simulink model "parity1"  (R2021b)
settings: Solver=ode45  StartTime=0.0  StopTime=30  RelTol=1e-3  EnableMultiTasking=on
undefined symbols (not defined in the file): A, B, C, D, Ef, Ff, Hus, Vs
settings Model: Creator=ak  LastModifiedBy=user
settings SolverCC: AlgebraicLoopSolver=TrustRegion
settings DataIOCC: LimitDataPoints=on  SaveFormat=Array  ReturnWorkspaceOutputs=off
settings OptimizationCC: ExpressionDepthLimit=2147483647  LifeSpan=inf
settings DebuggingCC: UnderspecifiedInitializationDetection=Classic  MergeDetectMultiDrivingBlocksExec=none  SolverPrmCheckMsg=warning  StateNameClashWarn=warning  SFUnexpectedBacktrackingDiag=warning  SFNoUnconditionalDefaultTransitionDiag=warning  SFExecutionAtInitializationDiag=none  SFMachineParentedDataDiag=warning  ArithmeticOperatorsInVariantConditions=warning
settings HardwareCC: ProdBitPerPointer=32  ProdBitPerSizeT=32  ProdBitPerPtrDiffT=32  ProdLargestAtomicFloat=None  ProdIntDivRoundTo=Undefined  ProdEndianess=Unspecified  ProdWordSize=32  ProdHWDeviceType=32-bit Generic
settings ModelReferenceCC: PropagateSignalLabelsOutOfModel=off
settings SFSimCC: SimUseLocalCustomCode=off  CustomCodeUndefinedFunction=UseInterfaceOnly
settings RTWCC: RTWUseLocalCustomCode=off
settings CodeAppCC: StateflowObjectComments=on
settings GRTTargetCC: TargetLangStandard=C89/C90 (ANSI)
settings ConfigComp: CovMetricSettings=dw  CovSaveCumulativeToWorkspaceVar=on  CovSaveSingleToWorkspaceVar=on  CovExternalEMLEnable=off

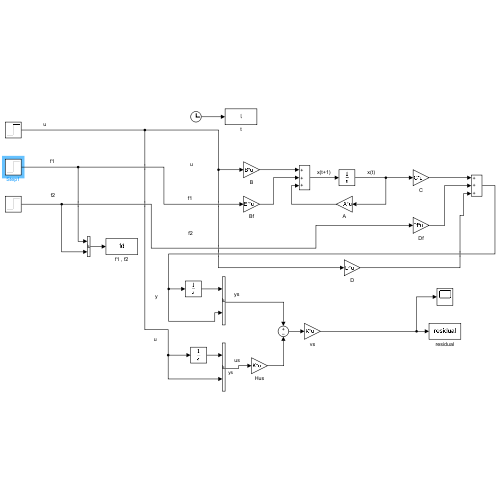
[thumbnail: Simulink's stored preview of the top-level diagram]
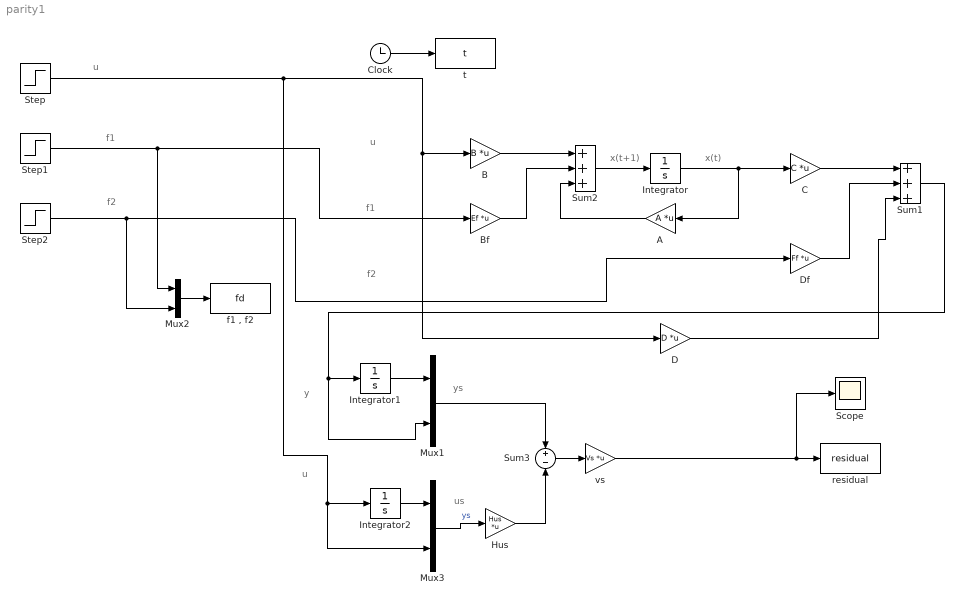
== system parity1 ==
  note: f2
  note: f1
  note: u
  note: x(t+1)
  note: f2
  note: f1
  note: x(t)
  note: u
  note: us
  note: ys
  note: y
  note: u
  A : Gain  Gain=A  Multiplication=Matrix(K*u)
  B : Gain  Gain=B  Multiplication=Matrix(K*u)
  Bf : Gain  Gain=Ef  Multiplication=Matrix(K*u)
  C : Gain  Gain=C  Multiplication=Matrix(K*u)
  Clock : Clock
  D : Gain  Gain=D  Multiplication=Matrix(K*u)
  Df : Gain  Gain=Ff  Multiplication=Matrix(K*u)
  Hus : Gain  Gain=Hus  Multiplication=Matrix(K*u)  SampleTime=.1
  Integrator : Integrator
  Integrator1 : Integrator
  Integrator2 : Integrator
  Mux1 : Mux  Inputs=2
  Mux2 : Mux  Inputs=2
  Mux3 : Mux  Inputs=2
  Scope : Scope
  Step : Step  Time=0  After=[1,1]  SampleTime=0
  Step1 : Step  After=[1,1,1]  SampleTime=0
  Step2 : Step  After=[1,1,1,1]  SampleTime=0
  Sum1 : Sum  Inputs=+++
  Sum2 : Sum  Inputs=+++
  Sum3 : Sum  Inputs=+-  SampleTime=.1
  "f1 , f2" : ToWorkspace  VariableName=fd  SampleTime=.01
  residual : ToWorkspace  VariableName=residual  SampleTime=.01
  t : ToWorkspace  VariableName=t  SampleTime=.01
  vs : Gain  Gain=Vs  Multiplication=Matrix(K*u)  SampleTime=.1
  wires:
  Clock/1 -> t/1
  vs/1 -> residual/1, Scope/1
  Mux2/1 -> "f1 , f2"/1
  A/1 -> Sum2/3
  D/1 -> Sum1/3
  Step1/1 -> Bf/1, Mux2/1
  Step2/1 -> Df/1, Mux2/2
  B/1 -> Sum2/1
  Bf/1 -> Sum2/2
  Integrator/1 -> C/1, A/1
  C/1 -> Sum1/1
  Df/1 -> Sum1/2
  Sum2/1 -> Integrator/1
  Mux3/1 -> Hus/1  "ys"
  Sum1/1 -> Integrator1/1, Mux1/2
  Sum3/1 -> vs/1
  Hus/1 -> Sum3/2
  Integrator1/1 -> Mux1/1
  Mux1/1 -> Sum3/1
  Step/1 -> Integrator2/1, Mux3/2, D/1, B/1
  Integrator2/1 -> Mux3/1
